simulink model "power_PVarray_islanding_detection"  (R2020a)
settings: Solver=VariableStepAuto  StartTime=0.0  StopTime=Simulation_Time  RelTol=1e-3
values from neighbouring files (symbols this model uses):
  Dinit = 0.5    [power_PVarray_100kW_param.m]
  Fnom = 60    [power_PVarray_100kW_param.m]
  Increment_MPPT = 0.01    [power_PVarray_100kW_param.m]
  Limits_MPPT = [ 1 0 ]    [power_PVarray_100kW_param.m]
  Pnom = 100e3    (= 100000)    [power_PVarray_100kW_param.m]
  Ts_Control = 10*Ts_Power    (= 5.05050505051e-05)    [power_PVarray_100kW_param.m]
  Ts_Power = 1/(33*Fnom)/100    (= 5.05050505051e-06)    [power_PVarray_100kW_param.m]
undefined symbols (not defined in the file or in its folder): D1, Delta
libraries: powerlib x29, powerlib_meascontrol x14, simulink x2, re_lib x1
(part 1 of 2)
settings Model: Creator=jfgf1  LastModifiedBy=jfgf1
settings DataIOCC: ReturnWorkspaceOutputs=off

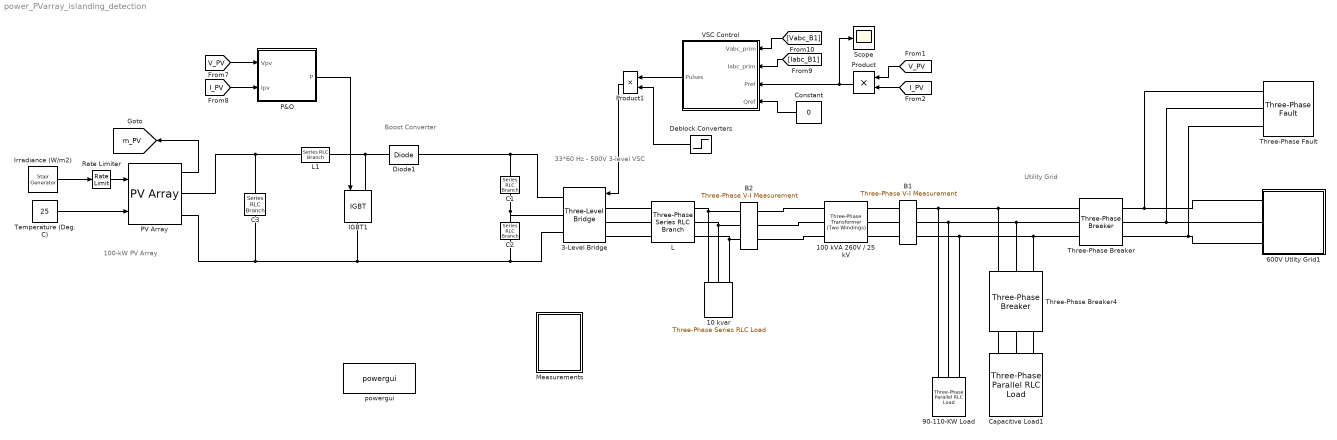
== system power_PVarray_islanding_detection ==
  note: Boost Converter
  note: 33*60 Hz - 500V
      | 3-level VSC
  note: 100-kW PV Array
  note: Utility Grid
  10 kvar : powerlib/Elements/Three-Phase Series RLC Load  LConnTagsString=A|B|C  Configuration=Y (grounded)  NominalVoltage=Vnom_dc  Vabc=[1e3 1e3 1e3]  Vabcp=[1e3 1e3 1e3]  NominalFrequency=Fnom  UnbalancedPower=off  ActivePower=10e3/100  InductivePower=0  CapacitivePower=10e3  Pabc=[10e3 9e3 11e3]  QLabc=[100 90 110]  QCabc=[100 90 110]  Pabcp=[10e3 9e3 11e3]  QLabcp=[100 90 110]  QCabcp=[100 90 110]  Measurements=None  LoadType=constant Z
  100 kVA 260V / 25 kV : powerlib/Elements/Three-Phase Transformer (Two Windings)  Winding1Connection=Yg  Winding2Connection=Delta (D1)  CoreType=Three single-phase transformers  SetSaturation=off  Hysteresis=off  DataFile='hysteresis'  SetInitialFlux=off  Measurements=None  UNITS=pu  NominalPower=[100e3 , 60 ]  Winding1=[ 25e3 , 0.001 , 0.03 ]  Winding2=[ 260 , 0.001 , 0.03 ]  Rm=500  Lm=500  L0=0.5  Saturation=[ 0,0 ; 0.0024,1.2 ; 1.0,1.52 ]  InitialFluxes=[ 0.8 , -0.8 , 0.7 ]  BreakLoop=off  DiscreteSolver=Trapezoidal iterative  DataType=off  TransfoNumber=0
  3-Level Bridge : powerlib/Power Electronics/Three-Level Bridge  Arms=3  SnubberResistance=1e6  SbubberCapacitance=inf  Device=IGBT / Diodes  Ron=0.2e-3  ForwardVoltages="[  0  0 ]"  Measurements=None
      settings: SourceProductBaseCode=PS
  600V Utlity Grid1 : Subsystem
      mask Display: image(imread('grid.jpg'))
  90-110-KW Load : powerlib/Elements/Three-Phase Parallel RLC Load  LConnTagsString=A|B|C  Configuration=Y (grounded)  NominalVoltage=Vnom_prim  Vabc=[1e3 1e3 1e3]  Vabcp=[1e3 1e3 1e3]  NominalFrequency=Fnom  UnbalancedPower=off  ActivePower=activeP  InductivePower=0  CapacitivePower=0  Pabc=[10e3 9e3 11e3]  QLabc=[100 90 110]  QCabc=[100 90 110]  Pabcp=[10e3 9e3 11e3]  QLabcp=[100 90 110]  QCabcp=[100 90 110]  Measurements=None  LoadType=constant Z
  B1 : powerlib/Measurements/Three-Phase V-I Measurement  VoltageMeasurement=phase-to-ground  SetLabelV=on  LabelV=Vabc_B1  Vpu=off  VpuLL=off  CurrentMeasurement=yes  SetLabelI=on  LabelI=Iabc_B1  Ipu=off  Pbase=100e6  Vbase=500e3  OutputType=Magnitude  PhasorSimulation=off  PSBequivalent=0
  B2 : powerlib/Measurements/Three-Phase V-I Measurement  VoltageMeasurement=phase-to-ground  SetLabelV=on  LabelV=Vabc  Vpu=off  VpuLL=off  CurrentMeasurement=no  SetLabelI=off  LabelI=Iabc  Ipu=off  Pbase=100e6  Vbase=500e3  OutputType=Magnitude  PhasorSimulation=off  PSBequivalent=0
  C1 : powerlib/Elements/Series RLC Branch  LConnTagsString=__new0  RConnTagsString=__new0  BranchType=C  Resistance=1.0  Inductance=1.0  SetiL0=off  InitialCurrent=0  Capacitance=12000e-06  Setx0=off  InitialVoltage=0  Measurements=None
  C2 : powerlib/Elements/Series RLC Branch  LConnTagsString=__new0  RConnTagsString=__new0  BranchType=C  Resistance=1.0  Inductance=1.0  SetiL0=off  InitialCurrent=0  Capacitance=12000e-06  Setx0=off  InitialVoltage=0  Measurements=None
  C3 : powerlib/Elements/Series RLC Branch  LConnTagsString=__new0  RConnTagsString=__new0  BranchType=C  Resistance=1.0  Inductance=1.0  SetiL0=off  InitialCurrent=0  Capacitance=100e-6  Setx0=off  InitialVoltage=0  Measurements=Branch voltage
  Capacitive Load1 : powerlib/Elements/Three-Phase Parallel RLC Load  LConnTagsString=A|B|C  Configuration=Y (grounded)  NominalVoltage=Vnom_prim  Vabc=[1e3 1e3 1e3]  Vabcp=[1e3 1e3 1e3]  NominalFrequency=Fnom  UnbalancedPower=off  ActivePower=0  InductivePower=0  CapacitivePower=800e3  Pabc=[10e3 9e3 11e3]  QLabc=[100 90 110]  QCabc=[100 90 110]  Pabcp=[10e3 9e3 11e3]  QLabcp=[100 90 110]  QCabcp=[100 90 110]  Measurements=None  LoadType=constant Z
  Constant : Constant  Value=0
  Deblock Converters : Step  Time=0.05  SampleTime=0
  Diode1 : powerlib/Power Electronics/Diode  Ron=1e-4  Lon=0  Vf=0  IC=0  UseSnubber=off  Rs=inf  Cs=inf  Measurements=off
  IGBT1 : powerlib/Power Electronics/IGBT  Ron=0.001  Lon=0  Vf=0  Tf=0  Tt=0  IC=0  Rs=1e5  Cs=inf  Measurements=off
  Irradiance (W/m2) : powerlib_meascontrol/Pulse & Signal Generators/Stair Generator  t=[0, 0.4, 1.0]  e=[1, 1, 1]*1000  Ts=Ts_Power
  L : powerlib/Elements/Three-Phase Series RLC Branch  LConnTagsString=A|B|C  RConnTagsString=A|B|C  BranchType=RL  Resistance=500e-6*377/50/2  Inductance=500e-6/2  Capacitance=inf  Measurements=None
  L1 : powerlib/Elements/Series RLC Branch  LConnTagsString=__new0  RConnTagsString=__new0  BranchType=RL  Resistance=0.005  Inductance=5e-3  SetiL0=off  InitialCurrent=0  Capacitance=1e-6  Setx0=off  InitialVoltage=0  Measurements=None
  Measurements : Subsystem
  P&O : Subsystem
  PV Array : re_lib/Solar/PV Array  Npar=66  Nser=5  PlotType=array @ 1000 W/m2 & specified temperatures  S_vec="[ 1000  250 ]"  Temp_C_vec="[0 25 50  ]"  ModuleName=SunPower SPR-305E-WHT-D  PlotWhenSelected=off  Pm=305.226  Ncell=96  Voc=64.2  Isc=5.96  Vm=54.7  Im=5.58  beta_Voc_pc=-0.27269  alpha_Isc_pc=0.061745  beta_Voc=-0.17507  alpha_Isc=0.00368  IL=6.0092  I0=6.3014e-12  nI=0.94504  Rsh=269.5934  Rs=0.37152  RobustModel=off  RobustCellTemperature=25  BAL=on  Tc=1e-6  Tfilter=5e-5
  Product : Product
  Product1 : Product  RndMeth=Zero
  Rate Limiter : RateLimiter  RisingSlewLimit=6000  FallingSlewLimit=-6000  SampleTimeMode=inherited  InitialCondition=1000
  Scope : Scope
  Temperature (Deg. C) : Constant  Value=25
  Three-Phase Breaker : powerlib/Elements/Three-Phase Breaker  InitialState=closed  SwitchA=on  SwitchB=on  SwitchC=on  SwitchTimes=switching_PCC  External=off  BreakerResistance=0.01  SnubberResistance=1e6  SnubberCapacitance=inf  Measurements=None
  Three-Phase Breaker4 : powerlib/Elements/Three-Phase Breaker  InitialState=closed  SwitchA=on  SwitchB=on  SwitchC=on  SwitchTimes=switching_C  External=off  BreakerResistance=0.01  SnubberResistance=800e3  SnubberCapacitance=inf  Measurements=None
  Three-Phase Fault : powerlib/Elements/Three-Phase Fault  InitialStates=0  FaultA=on  FaultB=off  FaultC=off  GroundFault=on  SwitchTimes=switching_fault  External=off  SwitchStatus=NaN  FaultResistance=0.001  GroundResistance=0.01  SnubberResistance=1e6  SnubberCapacitance=inf  Measurements=None
  VSC Control : Subsystem  mask(VSC Main Controller){nom=[ Pnom  Fnom ], Vnom=[ 25e3 260 ], Vnom_dc=500, RLxfo=[0.002  0.06 ], RLchoke=[2e-3  250e-6  ], K_VDCreg=[7  800], K_Ireg=[0.3 20], Ts=Ts_Control}
      mask prompts: nom "Nominal power and frequency [ Pnom(VA)  Fnom(Hz) ]:"; Vnom "Nominal primary and secondary voltages (Vrms LL) [ Vnom_prim   Vnom_sec ]:"; Vnom_dc "Nominal DC bus voltage (V):"; RLxfo "Total transformer leakage impedance (pu/Pnom) [ Rxfo  Lxf ]"; RLchoke "Choke impedance [ R(ohm) L(H) ]"; K_VDCreg "VDC regultator gains [ Kp  Ki ]:"; K_Ireg "Current regulator gains [ Kp  Ki ]:"; Ts "Sample time"
      mask init:
      | Pnom=nom(1);
      | Fnom=nom(2);
      | Vnom_prim=Vnom(1);
      | Vnom_sec=Vnom(2);
      | Zbase=Vnom_sec^2/Pnom;
      | Rtot_pu=RLxfo(1) + RLchoke(1)/Zbase;
      | Ltot_pu=RLxfo(2) + RLchoke(2)/(Zbase/(2*pi*Fnom));
      | Kp_VDCreg=K_VDCreg(1);
      | Ki_VDCreg=K_VDCreg(2);
      | Kp_Ireg=K_Ireg(1);
      | Ki_Ireg=K_Ireg(2);
      | Vdc_ref=Vnom_dc;
      | % Used to determine initial value of Boost Control (MPPT)
      | assignin('base','Vdc_ref_Inv',Vdc_ref);
  powergui : powerlib/powergui  Priority=1  SimulationMode=Discrete  SampleTime=1e-06  frequency=60  Iterations=50  frequencyindice=0  Pbase=100e6  ErrMax=1e-4  UnitsV=kV  UnitsW=MW  buscounter=0  FunctionMessages=off  echomessages=off  EnableUseOfTLC=off  CurrentSourceSwitches=off  DisableSnubberDevices=off  DisableRonSwitches=off  DisableVfSwitches=off  DisplayEquations=off  AutomaticDiscreteSolvers=off  SolverType=Tustin/Backward Euler (TBE)  Interpol=off  ExternalGateDelay=off  methode=off  Ts=0  x0status=blocks  SPID=off  SwTol=0  HookPort=off  NonlinearTolerance=1e-8  nMaxIteration=10  ContinueOnMaxIteration=off  RestoreLinks=warning  ResistiveCurrentMeasurement=off  Frange=[0:2:500]  Ylog=off  Xlog=on  ShowGrid=off  save=off  variable=ZData  structure=0  ZoomFFT=on  StartTime=0.0  cycles=1  DisplayStyle=1  fundamental=60  FreqAxis=off  MaxFrequency=1000  frequencyindicesteady=1  RmsSteady=1  display=off
  tag scope: m_PV=global
  wires:
  Temperature (Deg. C)/1 -> PV Array/2
  Irradiance (W/m2)/1 -> Rate Limiter/1
  PV Array/1 -> [m_PV]
  [V_PV] -> P&O/1(Vpv)
  [I_PV] -> P&O/2(Ipv)
  Constant/1 -> VSC Control/4(Qref)
  [I_PV] -> Product/2
  [V_PV] -> Product/1
  Product1/1 -> 3-Level Bridge/1
  Product/1 -> VSC Control/3(Pref), Scope/1
  [Iabc_B1] -> VSC Control/2(Iabc_prim)
  [Vabc_B1] -> VSC Control/1(Vabc_prim)
  VSC Control/1(Pulses) -> Product1/1
  Deblock Converters/1 -> Product1/2
  Rate Limiter/1 -> PV Array/1
  P&O/1(P) -> IGBT1/1
  connections:
  C3/LConn1 -- L1/LConn1 -- PV Array/RConn1
  3-Level Bridge/RConn3 -- IGBT1/RConn1 -- C3/RConn1 -- PV Array/RConn2 -- C2/RConn1
  3-Level Bridge/RConn1 -- C1/LConn1 -- Diode1/RConn1
  C2/LConn1 -- 3-Level Bridge/RConn2 -- C1/RConn1
  L1/RConn1 -- IGBT1/LConn1 -- Diode1/LConn1
  L/RConn2 -- B2/LConn2 -- 10 kvar/LConn2
  L/RConn1 -- 10 kvar/LConn1 -- B2/LConn1
  B2/LConn3 -- L/RConn3 -- 10 kvar/LConn3
  L/LConn1 -- 3-Level Bridge/LConn1
  L/LConn2 -- 3-Level Bridge/LConn2
  L/LConn3 -- 3-Level Bridge/LConn3
  100 kVA 260V / 25 kV/RConn3 -- B2/RConn3
  Three-Phase Breaker/LConn3 -- Three-Phase Breaker4/LConn3 -- 90-110-KW Load/LConn3 -- B1/RConn3
  Three-Phase Breaker/LConn1 -- Three-Phase Breaker4/LConn1 -- 90-110-KW Load/LConn1 -- B1/RConn1
  100 kVA 260V / 25 kV/RConn1 -- B2/RConn1
  Three-Phase Breaker/LConn2 -- Three-Phase Breaker4/LConn2 -- 90-110-KW Load/LConn2 -- B1/RConn2
  B1/LConn3 -- 100 kVA 260V / 25 kV/LConn3
  B1/LConn2 -- 100 kVA 260V / 25 kV/LConn2
  100 kVA 260V / 25 kV/RConn2 -- B2/RConn2
  B1/LConn1 -- 100 kVA 260V / 25 kV/LConn1
  Three-Phase Breaker/RConn1 -- Three-Phase Fault/LConn1 -- 600V Utlity Grid1/LConn1
  Three-Phase Breaker/RConn2 -- Three-Phase Fault/LConn2 -- 600V Utlity Grid1/LConn2
  Three-Phase Breaker/RConn3 -- Three-Phase Fault/LConn3 -- 600V Utlity Grid1/LConn3
  Capacitive Load1/LConn1 -- Three-Phase Breaker4/RConn1
  Three-Phase Breaker4/RConn2 -- Capacitive Load1/LConn2
  Three-Phase Breaker4/RConn3 -- Capacitive Load1/LConn3

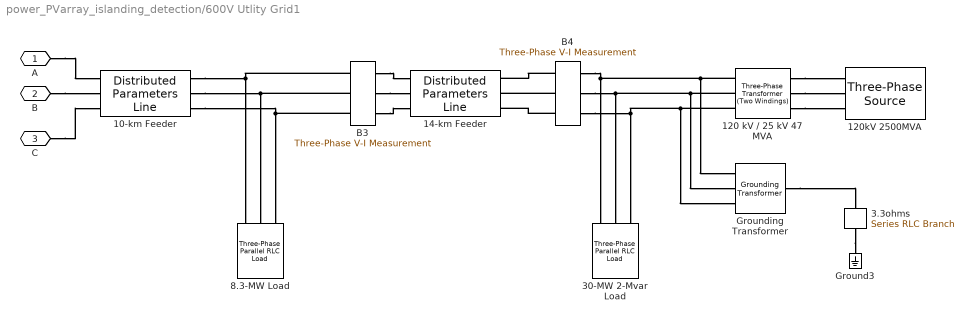
== system power_PVarray_islanding_detection/600V Utlity Grid1 ==
  10-km Feeder : powerlib/Elements/Distributed Parameters Line  Phases=3  Frequency=Fnom  Resistance=[0.1153 0.413]  Inductance=[1.05e-3 3.32e-3]  Capacitance=[11.33e-009 5.01e-009]  Length=10  x1=[-4.1e-05 1.31145391612596e-09 0 0;-4e-05 1.3127563025415e-09 0 0;-3.9e-05 1.31405850238509e-09 0 0;-3.8e-05 1.31536051547166e-09 0 0;-3.7e-05 1.31666234161617e-09 0 0;-3.6e-05 1.3179639806336e-09 0 0;-3.5e-05 1.31926543233895e-09 -5402.42576667042 -23138.0301536426;-3.4e-05 1.32056669654726e-09 -5393.70255110855 -23140.0651759113;-3.3e-05 1.3218677730736e-09 -5384.97856898125 -23142.0969094607;-3.2e-05 1.32316866173304e-09 -5376.2538215284 -23144.125354002;-3.1e-05 1.32446936234071e-09 -5367.52830998999 -23146.150509247;-3e-05 1.32576987471174e-09 -5358.8020356061 -23148.1723749077;-2.9e-05 1.32707019866131e-09 -5350.07499961693 -23150.190950697;-2.8e-05 1.32837033400461e-09 -5341.34720326278 -23152.2062363278;-2.7e-05 1.32967028055686e-09 -5332.61864778408 -23154.2182315137;-2.6e-05 1.3309700381333e-09 -5323.88933442134 -23156.2269359689;-2.5e-05 1.33226960654922e-09 -5315.1592644152 -23158.2323494078;-2.4e-05 1.33356898561992e-09 -5306.42843900638 -23160.2344715454;-2.3e-05 1.33486817516073e-09 -5297.69685943574 -23162.2333020972;-2.2e-05 1.33616717498699e-09 -5288.96452694423 -23164.2288407791;-2.1e-05 1.33746598491411e-09 -5280.23144277291 -23166.2210873075;-2e-05 1.33876460475747e-09 -5271.49760816295 -23168.2100413992;-1.9e-05 1.34006303433253e-09 -5262.76302435561 -23170.1957027716;-1.8e-05 1.34136127345475e-09 -5254.02769259227 -23172.1780711424;-1.7e-05 1.34265932193962e-09 -5245.29161411443 -23174.1571462299;-1.6e-05 1.34395717960265e-09 -5236.55479016367 -23176.1329277529;-1.5e-05 1.3452548462594e-09 -5227.81722198169 -23178.1054154305;-1.4e-05 1.34655232172543e-09 -5219.07891081029 -23180.0746089825;-1.3e-05 1.34784960581635e-09 -5210.33985789138 -23182.0405081288;-1.2e-05 1.34914669834777e-09 -5201.60006446699 -23184.0031125903;-1.1e-05 1.35044359913537e-09 -5192.85953177921 -23185.9624220878;-1e-05 1.35174030799481e-09 -5184.11826107029 -23187.918436343;-9e-06 1.3530368247418e-09 -5175.37625358255 -23189.8711550778;-8e-06 1.35433314919209e-09 -5166.63351055843 -23191.8205780148;-7e-06 1.35562928116144e-09 -5157.89003324046 -23193.7667048769;-6e-06 1.35692522046563e-09 -5149.14582287128 -23195.7095353875;-5e-06 1.35822096692048e-09 -5140.40088069365 -23197.6490692704;-4e-06 1.35951652034185e-09 -5131.65520795041 -23199.58530625;-3e-06 1.3608118805456e-09 -5122.90880588453 -23201.5182460512;-2e-06 1.36210704734763e-09 -5114.16167573905 -23203.4478883992;-1e-06 1.36340202056387e-09 -5105.41381875715 -23205.3742330198]  x2=[-4.1e-05 1.33995737415073e-09 0 0;-4e-05 1.34130776092081e-09 0 0;-3.9e-05 1.34265795706114e-09 0 0;-3.8e-05 1.34400796237984e-09 0 0;-3.7e-05 1.34535777668502e-09 0 0;-3.6e-05 1.34670739978487e-09 0 0;-3.5e-05 1.34805683148756e-09 -5385.24656512758 -23143.2120767652;-3.4e-05 1.34940607160131e-09 -5376.52139724753 -23145.2406222594;-3.3e-05 1.35075511993436e-09 -5367.79546524388 -23147.2658782988;-3.2e-05 1.35210397629498e-09 -5359.06877035679 -23149.2878445954;-3.1e-05 1.35345264049148e-09 -5350.34131382651 -23151.306520862;-3e-05 1.35480111233217e-09 -5341.61309689341 -23153.3219068116;-2.9e-05 1.35614939162541e-09 -5332.88412079796 -23155.3340021579;-2.8e-05 1.35749747817958e-09 -5324.15438678074 -23157.3428066147;-2.7e-05 1.35884537180308e-09 -5315.42389608245 -23159.3483198967;-2.6e-05 1.36019307230434e-09 -5306.69264994387 -23161.3505417188;-2.5e-05 1.36154057949184e-09 -5297.96064960593 -23163.3494717965;-2.4e-05 1.36288789317406e-09 -5289.22789630962 -23165.3451098456;-2.3e-05 1.36423501315951e-09 -5280.49439129607 -23167.3374555825;-2.2e-05 1.36558193925674e-09 -5271.7601358065 -23169.3265087242;-2.1e-05 1.36692867127433e-09 -5263.02513108225 -23171.3122689878;-2e-05 1.36827520902086e-09 -5254.28937836475 -23173.2947360912;-1.9e-05 1.36962155230498e-09 -5245.55287889556 -23175.2739097525;-1.8e-05 1.37096770093532e-09 -5236.81563391631 -23177.2497896907;-1.7e-05 1.37231365472058e-09 -5228.07764466877 -23179.2223756247;-1.6e-05 1.37365941346947e-09 -5219.33891239481 -23181.1916672743;-1.5e-05 1.37500497699072e-09 -5210.59943833638 -23183.1576643596;-1.4e-05 1.37635034509309e-09 -5201.85922373557 -23185.1203666012;-1.3e-05 1.37769551758539e-09 -5193.11826983455 -23187.07977372;-1.2e-05 1.37904049427643e-09 -5184.37657787562 -23189.0358854378;-1.1e-05 1.38038527497506e-09 -5175.63414910114 -23190.9887014764;-1e-05 1.38172985949015e-09 -5166.89098475364 -23192.9382215583;-9e-06 1.38307424763062e-09 -5158.14708607569 -23194.8844454064;-8e-06 1.38441843920539e-09 -5149.40245431 -23196.8273727442;-7e-06 1.38576243402343e-09 -5140.65709069939 -23198.7670032954;-6e-06 1.38710623189373e-09 -5131.91099648676 -23200.7033367845;-5e-06 1.38844983262529e-09 -5123.16417291513 -23202.6363729363;-4e-06 1.38979323602716e-09 -5114.41662122761 -23204.5661114759;-3e-06 1.39113644190842e-09 -5105.66834266743 -23206.4925521292;-2e-06 1.39247945007817e-09 -5096.91933847791 -23208.4156946224;-1e-06 1.39382226034554e-09 -5088.16960990249 -23210.3355386821]  x3=[-4.1e-05 -6.52349176014467e-12 0 0;-4e-05 -6.52032398932471e-12 0 0;-3.9e-05 -6.5171552918213e-12 0 0;-3.8e-05 -6.51398566808478e-12 0 0;-3.7e-05 -6.51081511856562e-12 0 0;-3.6e-05 -6.50764364371443e-12 0 0;-3.5e-05 -6.50447124398195e-12 -18.2306561580198 -80.0189566853611;-3.4e-05 -6.50129791981904e-12 -18.2004884272665 -80.0258237944139;-3.3e-05 -6.49812367167671e-12 -18.1703181098179 -80.0326795300124;-3.2e-05 -6.49494850000609e-12 -18.1401452099618 -80.0395238911823;-3.1e-05 -6.49177240525843e-12 -18.1099697319866 -80.0463568769508;-3e-05 -6.48859538788514e-12 -18.0797916801808 -80.0531784863469;-2.9e-05 -6.48541744833774e-12 -18.0496110588333 -80.0599887184009;-2.8e-05 -6.48223858706789e-12 -18.0194278722336 -80.0667875721451;-2.7e-05 -6.47905880452736e-12 -17.9892421246714 -80.0735750466132;-2.6e-05 -6.47587810116809e-12 -17.9590538204366 -80.0803511408404;-2.5e-05 -6.47269647744211e-12 -17.9288629638198 -80.0871158538639;-2.4e-05 -6.46951393380161e-12 -17.8986695591117 -80.0938691847221;-2.3e-05 -6.4663304706989e-12 -17.8684736106034 -80.1006111324552;-2.2e-05 -6.46314608858642e-12 -17.8382751225866 -80.1073416961052;-2.1e-05 -6.45996078791675e-12 -17.8080740993531 -80.1140608747153;-2e-05 -6.45677456914257e-12 -17.7778705451951 -80.1207686673307;-1.9e-05 -6.45358743271674e-12 -17.7476644644052 -80.1274650729981;-1.8e-05 -6.4503993790922e-12 -17.7174558612764 -80.1341500907657;-1.7e-05 -6.44721040872206e-12 -17.687244740102 -80.1408237196834;-1.6e-05 -6.44402052205953e-12 -17.6570311051756 -80.1474859588029;-1.5e-05 -6.44082971955798e-12 -17.6268149607914 -80.1541368071771;-1.4e-05 -6.43763800167088e-12 -17.5965963112436 -80.1607762638609;-1.3e-05 -6.43444536885185e-12 -17.566375160827 -80.1674043279107;-1.2e-05 -6.43125182155463e-12 -17.5361515138368 -80.1740209983845;-1.1e-05 -6.4280573602331e-12 -17.5059253745684 -80.1806262743419;-1e-05 -6.42486198534127e-12 -17.4756967473176 -80.1872201548441;-9e-06 -6.42166569733326e-12 -17.4454656363805 -80.193802638954;-8e-06 -6.41846849666335e-12 -17.4152320460537 -80.2003737257361;-7e-06 -6.41527038378591e-12 -17.384995980634 -80.2069334142565;-6e-06 -6.41207135915548e-12 -17.3547574444187 -80.2134817035829;-5e-06 -6.40887142322672e-12 -17.3245164417053 -80.2200185927847;-4e-06 -6.40567057645439e-12 -17.2942729767918 -80.2265440809328;-3e-06 -6.40246881929342e-12 -17.2640270539763 -80.2330581670998;-2e-06 -6.39926615219885e-12 -17.2337786775576 -80.2395608503598;-1e-06 -6.39606257562584e-12 -17.2035278518347 -80.2460521297888]  x4=[-4.1e-05 1.05357842266867e-11 0 0;-4e-05 1.05355469230034e-11 0 0;-3.9e-05 1.05353081219839e-11 0 0;-3.8e-05 1.05350678236622e-11 0 0;-3.7e-05 1.05348260280724e-11 0 0;-3.6e-05 1.05345827352489e-11 0 0;-3.5e-05 1.05343379452263e-11 -18.0916660851199 -71.3485155916182;-3.4e-05 1.05340916580393e-11 -18.0647670434512 -71.3553309187807;-3.3e-05 1.05338438737229e-11 -18.0378654343762 -71.3621361047593;-3.2e-05 1.05335945923124e-11 -18.0109612617182 -71.368931148587;-3.1e-05 1.05333438138432e-11 -17.984054529301 -71.3757160492978;-3e-05 1.05330915383509e-11 -17.9571452409485 -71.3824908059276;-2.9e-05 1.05328377658714e-11 -17.9302334004853 -71.3892554175135;-2.8e-05 1.05325824964408e-11 -17.903319011736 -71.3960098830941;-2.7e-05 1.05323257300953e-11 -17.8764020785258 -71.4027542017095;-2.6e-05 1.05320674668714e-11 -17.8494826046801 -71.409488372401;-2.5e-05 1.05318077068058e-11 -17.822560594025 -71.4162123942117;-2.4e-05 1.05315464499355e-11 -17.7956360503865 -71.422926266186;-2.3e-05 1.05312836962976e-11 -17.7687089775912 -71.4296299873696;-2.2e-05 1.05310194459294e-11 -17.7417793794661 -71.4363235568097;-2.1e-05 1.05307536988685e-11 -17.7148472598385 -71.4430069735551;-2e-05 1.05304864551526e-11 -17.6879126225361 -71.4496802366559;-1.9e-05 1.05302177148197e-11 -17.6609754713868 -71.4563433451637;-1.8e-05 1.05299474779081e-11 -17.634035810219 -71.4629962981316;-1.7e-05 1.05296757444561e-11 -17.6070936428614 -71.4696390946139;-1.6e-05 1.05294025145023e-11 -17.5801489731432 -71.4762717336666;-1.5e-05 1.05291277880857e-11 -17.5532018048937 -71.482894214347;-1.4e-05 1.05288515652451e-11 -17.5262521419428 -71.489506535714;-1.3e-05 1.05285738460199e-11 -17.4992999881206 -71.4961086968278;-1.2e-05 1.05282946304496e-11 -17.4723453472576 -71.50270069675;-1.1e-05 1.05280139185738e-11 -17.4453882231846 -71.5092825345439;-1e-05 1.05277317104325e-11 -17.418428619733 -71.5158542092739;-9e-06 1.05274480060657e-11 -17.3914665407341 -71.5224157200061;-8e-06 1.05271628055137e-11 -17.36450199002 -71.5289670658079;-7e-06 1.05268761088171e-11 -17.337534971423 -71.5355082457484;-6e-06 1.05265879160167e-11 -17.3105654887755 -71.5420392588977;-5e-06 1.05262982271534e-11 -17.2835935459107 -71.5485601043278;-4e-06 1.05260070422683e-11 -17.2566191466617 -71.5550707811118;-3e-06 1.05257143614029e-11 -17.2296422948623 -71.5615712883244;-2e-06 1.05254201845987e-11 -17.2026629943465 -71.5680616250419;-1e-06 1.05251245118976e-11 -17.1756812489486 -71.5745417903416]  x5=4.0783820321299e-05  V1=[0 0 0 7.655e-09 2.411e+04 2.411e+04;0 0 0 377 377 377;1.571 1.571 1.571 -2.646 -0.2338 -1.805]  V2=[0 0 0 7.796e-09 2.399e+04 2.399e+04;0 0 0 377 377 377;1.571 1.571 1.571 -2.649 -0.2317 -1.803]  I1=[0 0 0 1.571e-11 88.21 88.21;0 0 0 377 377 377;1.571 1.571 1.571 2.839 0.1284 -1.442]  I2=[0 0 0 1.332e-11 81.66 81.66;0 0 0 377 377 377;1.571 1.571 1.571 -1.715 -0.638 -2.209]  nHarmo=2  Measurements=None
  120 kV / 25 kV 47 MVA : powerlib/Elements/Three-Phase Transformer (Two Windings)  Winding1Connection=Yg  Winding2Connection=Delta (D1)  CoreType=Three single-phase transformers  SetSaturation=off  Hysteresis=off  DataFile='basic_model'  SetInitialFlux=off  Measurements=None  UNITS=pu  NominalPower=[47e6 60 ]  Winding1="[ 120e3  0.08/30   0.08 ]"  Winding2="[ 25e3  0.08/30  0.08]"  Rm=500  Lm=500  L0=0.5  Saturation="[ 0,0  ;  0.005,1.2  ;  1.0,1.4 ]"  InitialFluxes=[ 0.8 , -0.8 , 0.7 ]  BreakLoop=off  DiscreteSolver=Trapezoidal iterative  DataType=off  TransfoNumber=0
  120kV 2500MVA : powerlib/Electrical Sources/Three-Phase Source  InternalConnection=Yg  VoltagePhases=off  Voltage=120e3  PhaseAngle=0  Voltage_phases=[25e3 25e3 25e3]/sqrt(3)  PhaseAngles_phases=[0 -120 +120]  Frequency=Fnom  NonIdealSource=on  SpecifyImpedance=on  Resistance=0.8929  Inductance=16.58e-3  ShortCircuitLevel=2500e6  BaseVoltage=120e3  XRratio=7  BusType=swing  Pref=0  Qref=0  Prefabc=[10e3, 10e3, 10e3]  Qrefabc=[0, 0, 0]  Qmin=-inf  Qmax=inf
  14-km Feeder : powerlib/Elements/Distributed Parameters Line  Phases=3  Frequency=Fnom  Resistance=[0.1153 0.413]  Inductance=[1.05e-3 3.32e-3]  Capacitance=[11.33e-009 5.01e-009]  Length=14  x1=[-5.8e-05 1.31605259900835e-09 0 0;-5.7e-05 1.31740636106194e-09 0 0;-5.6e-05 1.3187599358827e-09 0 0;-5.5e-05 1.32011332327827e-09 0 0;-5.4e-05 1.32146652305629e-09 0 0;-5.3e-05 1.32281953502445e-09 0 0;-5.2e-05 1.32417235899045e-09 0 0;-5.1e-05 1.32552499476203e-09 0 0;-5e-05 1.32687744214694e-09 0 0;-4.9e-05 1.32822970095298e-09 -5507.3179882465 -23114.4672093839;-4.8e-05 1.32958177098796e-09 -5498.60364825136 -23116.541776762;-4.7e-05 1.33093365205971e-09 -5489.88852678202 -23118.613058764;-4.6e-05 1.33228534397611e-09 -5481.17262507708 -23120.6810550955;-4.5e-05 1.33363684654505e-09 -5472.45594437527 -23122.7457654626;-4.4e-05 1.33498815957446e-09 -5463.73848591543 -23124.8071895718;-4.3e-05 1.33633928287227e-09 -5455.02025093649 -23126.8653271303;-4.2e-05 1.33769021624647e-09 -5446.30124067753 -23128.9201778453;-4.1e-05 1.33904095950505e-09 -5437.58145637769 -23130.9717414251;-4e-05 1.34039151245606e-09 -5428.86089927627 -23133.0200175778;-3.9e-05 1.34174187490753e-09 -5420.13957061263 -23135.0650060125;-3.8e-05 1.34309204666756e-09 -5411.41747162629 -23137.1067064386;-3.7e-05 1.34444202754426e-09 -5402.69460355684 -23139.1451185657;-3.6e-05 1.34579181734577e-09 -5393.97096764399 -23141.1802421044;-3.5e-05 1.34714141588024e-09 -5385.24656512758 -23143.2120767652;-3.4e-05 1.34849082295587e-09 -5376.52139724753 -23145.2406222594;-3.3e-05 1.34984003838089e-09 -5367.79546524388 -23147.2658782988;-3.2e-05 1.35118906196353e-09 -5359.06877035679 -23149.2878445954;-3.1e-05 1.35253789351207e-09 -5350.34131382651 -23151.306520862;-3e-05 1.35388653283481e-09 -5341.61309689341 -23153.3219068116;-2.9e-05 1.35523497974009e-09 -5332.88412079796 -23155.3340021579;-2.8e-05 1.35658323403624e-09 -5324.15438678074 -23157.3428066147;-2.7e-05 1.35793129553167e-09 -5315.42389608245 -23159.3483198967;-2.6e-05 1.35927916403478e-09 -5306.69264994387 -23161.3505417188;-2.5e-05 1.360626839354e-09 -5297.96064960593 -23163.3494717965;-2.4e-05 1.3619743212978e-09 -5289.22789630962 -23165.3451098456;-2.3e-05 1.36332160967468e-09 -5280.49439129607 -23167.3374555825;-2.2e-05 1.36466870429315e-09 -5271.7601358065 -23169.3265087242;-2.1e-05 1.36601560496177e-09 -5263.02513108225 -23171.3122689878;-2e-05 1.3673623114891e-09 -5254.28937836475 -23173.2947360912;-1.9e-05 1.36870882368376e-09 -5245.55287889556 -23175.2739097525;-1.8e-05 1.37005514135436e-09 -5236.81563391631 -23177.2497896907;-1.7e-05 1.37140126430958e-09 -5228.07764466877 -23179.2223756247;-1.6e-05 1.37274719235809e-09 -5219.33891239481 -23181.1916672743;-1.5e-05 1.37409292530862e-09 -5210.59943833638 -23183.1576643596;-1.4e-05 1.37543846296989e-09 -5201.85922373557 -23185.1203666012;-1.3e-05 1.37678380515068e-09 -5193.11826983455 -23187.07977372;-1.2e-05 1.37812895165979e-09 -5184.37657787562 -23189.0358854378;-1.1e-05 1.37947390230604e-09 -5175.63414910114 -23190.9887014764;-1e-05 1.38081865689828e-09 -5166.89098475364 -23192.9382215583;-9e-06 1.3821632152454e-09 -5158.14708607569 -23194.8844454064;-8e-06 1.3835075771563e-09 -5149.40245431 -23196.8273727442;-7e-06 1.38485174243992e-09 -5140.65709069939 -23198.7670032954;-6e-06 1.38619571090522e-09 -5131.91099648676 -23200.7033367845;-5e-06 1.3875394823612e-09 -5123.16417291513 -23202.6363729363;-4e-06 1.38888305661687e-09 -5114.41662122761 -23204.5661114759;-3e-06 1.39022643348129e-09 -5105.66834266743 -23206.4925521292;-2e-06 1.39156961276353e-09 -5096.91933847791 -23208.4156946224;-1e-06 1.39291259427268e-09 -5088.16960990249 -23210.3355386821]  x2=[-5.8e-05 2.25260683526935e-09 0 0;-5.7e-05 2.25401532245857e-09 0 0;-5.6e-05 2.25542348930195e-09 0 0;-5.5e-05 2.25683133559935e-09 0 0;-5.4e-05 2.25823886115068e-09 0 0;-5.3e-05 2.25964606575591e-09 0 0;-5.2e-05 2.26105294921504e-09 0 0;-5.1e-05 2.26245951132812e-09 0 0;-5e-05 2.26386575189524e-09 0 0;-4.9e-05 2.26527167071656e-09 -3896.85585223855 -24016.4611431425;-4.8e-05 2.26667726759225e-09 -3887.80158299085 -24017.9285165165;-4.7e-05 2.26808254232255e-09 -3878.74676119984 -24019.3924764071;-4.6e-05 2.26948749470774e-09 -3869.69138815242 -24020.8530226064;-4.5e-05 2.27089212454814e-09 -3860.63546513555 -24022.3101549068;-4.4e-05 2.27229643164413e-09 -3851.57899343628 -24023.7638731012;-4.3e-05 2.27370041579612e-09 -3842.52197434174 -24025.2141769829;-4.2e-05 2.27510407680457e-09 -3833.46440913913 -24026.661066346;-4.1e-05 2.27650741446999e-09 -3824.40629911574 -24028.1045409846;-4e-05 2.27791042859294e-09 -3815.34764555892 -24029.5446006937;-3.9e-05 2.27931311897402e-09 -3806.28844975611 -24030.9812452687;-3.8e-05 2.28071548541387e-09 -3797.22871299482 -24032.4144745052;-3.7e-05 2.28211752771319e-09 -3788.16843656266 -24033.8442881997;-3.6e-05 2.28351924567271e-09 -3779.10762174727 -24035.270686149;-3.5e-05 2.28492063909322e-09 -3770.04626983641 -24036.6936681502;-3.4e-05 2.28632170777554e-09 -3760.9843821179 -24038.1132340012;-3.3e-05 2.28772245152057e-09 -3751.92195987963 -24039.5293835003;-3.2e-05 2.28912287012921e-09 -3742.85900440957 -24040.9421164461;-3.1e-05 2.29052296340245e-09 -3733.79551699578 -24042.3514326378;-3e-05 2.29192273114129e-09 -3724.73149892638 -24043.7573318753;-2.9e-05 2.29332217314679e-09 -3715.66695148956 -24045.1598139586;-2.8e-05 2.29472128922007e-09 -3706.6018759736 -24046.5588786884;-2.7e-05 2.29612007916228e-09 -3697.53627366686 -24047.954525866;-2.6e-05 2.29751854277461e-09 -3688.47014585774 -24049.3467552929;-2.5e-05 2.29891667985832e-09 -3679.40349383476 -24050.7355667713;-2.4e-05 2.30031449021471e-09 -3670.33631888649 -24052.1209601038;-2.3e-05 2.3017119736451e-09 -3661.26862230157 -24053.5029350935;-2.2e-05 2.30310912995089e-09 -3652.20040536873 -24054.881491544;-2.1e-05 2.30450595893351e-09 -3643.13166937676 -24056.2566292593;-2e-05 2.30590246039444e-09 -3634.06241561453 -24057.6283480442;-1.9e-05 2.3072986341352e-09 -3624.99264537098 -24058.9966477035;-1.8e-05 2.30869447995737e-09 -3615.92235993514 -24060.3615280428;-1.7e-05 2.31008999766257e-09 -3606.85156059609 -24061.7229888681;-1.6e-05 2.31148518705245e-09 -3597.78024864299 -24063.081029986;-1.5e-05 2.31288004792875e-09 -3588.70842536509 -24064.4356512035;-1.4e-05 2.31427458009321e-09 -3579.63609205168 -24065.7868523279;-1.3e-05 2.31566878334763e-09 -3570.56324999215 -24067.1346331674;-1.2e-05 2.31706265749388e-09 -3561.48990047595 -24068.4789935303;-1.1e-05 2.31845620233386e-09 -3552.41604479262 -24069.8199332255;-1e-05 2.3198494176695e-09 -3543.34168423173 -24071.1574520625;-9e-06 2.3212423033028e-09 -3534.26682008297 -24072.4915498512;-8e-06 2.3226348590358e-09 -3525.19145363608 -24073.8222264021;-7e-06 2.32402708467059e-09 -3516.11558618086 -24075.1494815259;-6e-06 2.3254189800093e-09 -3507.0392190072 -24076.473315034;-5e-06 2.32681054485412e-09 -3497.96235340506 -24077.7937267383;-4e-06 2.32820177900726e-09 -3488.88499066446 -24079.1107164512;-3e-06 2.32959268227101e-09 -3479.80713207549 -24080.4242839854;-2e-06 2.33098325444769e-09 -3470.72877892832 -24081.7344291543;-1e-06 2.33237349533965e-09 -3461.64993251319 -24083.0411517717]  x3=[-5.8e-05 9.77969712792975e-12 0 0;-5.7e-05 9.80058033689096e-12 0 0;-5.6e-05 9.82146215297113e-12 0 0;-5.5e-05 9.8423425732025e-12 0 0;-5.4e-05 9.86322159461749e-12 0 0;-5.3e-05 9.88409921424873e-12 0 0;-5.2e-05 9.90497542912903e-12 0 0;-5.1e-05 9.92585023629143e-12 0 0;-5e-05 9.94672363276914e-12 0 0;-4.9e-05 9.9675956155956e-12 -90.5346088964957 -386.232113122669;-4.8e-05 9.98846618180443e-12 -90.3889963901512 -386.266216419227;-4.7e-05 1.00093353284295e-11 -90.2433710375146 -386.30026481874;-4.6e-05 1.00302030525047e-11 -90.0977328592823 -386.334258316372;-4.5e-05 1.00510693510644e-11 -89.9520818761529 -386.368196907289;-4.4e-05 1.0071934221143e-11 -89.8064181088265 -386.402080586668;-4.3e-05 1.00927976597751e-11 -89.6607415780053 -386.435909349695;-4.2e-05 1.01136596639956e-11 -89.5150523043932 -386.469683191561;-4.1e-05 1.01345202308395e-11 -89.3693503086958 -386.503402107465;-4e-05 1.0155379357342e-11 -89.2236356116206 -386.537066092617;-3.9e-05 1.01762370405387e-11 -89.0779082338769 -386.570675142231;-3.8e-05 1.01970932774651e-11 -88.9321681961759 -386.604229251531;-3.7e-05 1.02179480651572e-11 -88.7864155192305 -386.637728415748;-3.6e-05 1.0238801400651e-11 -88.6406502237553 -386.671172630122;-3.5e-05 1.02596532809827e-11 -88.4948723304669 -386.704561889898;-3.4e-05 1.02805037031889e-11 -88.3490818600835 -386.737896190332;-3.3e-05 1.03013526643063e-11 -88.2032788333253 -386.771175526685;-3.2e-05 1.03222001613717e-11 -88.0574632709141 -386.80439989423;-3.1e-05 1.03430461914223e-11 -87.9116351935735 -386.837569288242;-3e-05 1.03638907514953e-11 -87.765794622029 -386.870683704009;-2.9e-05 1.03847338386283e-11 -87.6199415770077 -386.903743136824;-2.8e-05 1.04055754498591e-11 -87.4740760792387 -386.936747581988;-2.7e-05 1.04264155822255e-11 -87.3281981494526 -386.969697034811;-2.6e-05 1.04472542327657e-11 -87.182307808382 -387.00259149061;-2.5e-05 1.04680913985181e-11 -87.0364050767612 -387.03543094471;-2.4e-05 1.04889270765213e-11 -86.8904899753261 -387.068215392444;-2.3e-05 1.0509761263814e-11 -86.7445625248146 -387.100944829152;-2.2e-05 1.05305939574353e-11 -86.5986227459662 -387.133619250182;-2.1e-05 1.05514251544243e-11 -86.4526706595223 -387.166238650892;-2e-05 1.05722548518204e-11 -86.3067062862258 -387.198803026645;-1.9e-05 1.05930830466634e-11 -86.1607296468215 -387.231312372812;-1.8e-05 1.06139097359931e-11 -86.014740762056 -387.263766684775;-1.7e-05 1.06347349168494e-11 -85.8687396526776 -387.296165957919;-1.6e-05 1.06555585862728e-11 -85.7227263394363 -387.328510187641;-1.5e-05 1.06763807413036e-11 -85.5767008430838 -387.360799369343;-1.4e-05 1.06972013789826e-11 -85.4306631843736 -387.393033498437;-1.3e-05 1.07180204963508e-11 -85.2846133840609 -387.425212570342;-1.2e-05 1.07388380904492e-11 -85.1385514629027 -387.457336580483;-1.1e-05 1.07596541583192e-11 -84.9924774416575 -387.489405524296;-1e-05 1.07804686970024e-11 -84.8463913410858 -387.521419397223;-9e-06 1.08012817035406e-11 -84.7002931819498 -387.553378194714;-8e-06 1.08220931749757e-11 -84.5541829850131 -387.585281912227;-7e-06 1.08429031083501e-11 -84.4080607710412 -387.617130545227;-6e-06 1.08637115007061e-11 -84.2619265608016 -387.648924089188;-5e-06 1.08845183490865e-11 -84.1157803750629 -387.680662539593;-4e-06 1.0905323650534e-11 -83.969622234596 -387.712345891929;-3e-06 1.09261274020919e-11 -83.823452160173 -387.743974141694;-2e-06 1.09469296008033e-11 -83.6772701725682 -387.775547284393;-1e-06 1.0967730243712e-11 -83.531076292557 -387.807065315538]  x4=[-5.8e-05 -5.22013038447485e-12 0 0;-5.7e-05 -5.2375749695159e-12 0 0;-5.6e-05 -5.25501881018074e-12 0 0;-5.5e-05 -5.27246190399021e-12 0 0;-5.4e-05 -5.28990424846526e-12 0 0;-5.3e-05 -5.30734584112694e-12 0 0;-5.2e-05 -5.32478667949642e-12 0 0;-5.1e-05 -5.34222676109495e-12 0 0;-5e-05 -5.35966608344392e-12 0 0;-4.9e-05 -5.37710464406482e-12 58.360070334798 232.30717909782;-4.8e-05 -5.39454244047922e-12 58.2724884464711 232.329163817471;-4.7e-05 -5.41197947020884e-12 58.1848982763241 232.351115517966;-4.6e-05 -5.42941573077547e-12 58.0972998368054 232.373034196185;-4.5e-05 -5.44685121970105e-12 58.0096931403648 232.394919849015;-4.4e-05 -5.46428593450759e-12 57.922078199453 232.416772473343;-4.3e-05 -5.48171987271724e-12 57.8344550265221 232.438592066065;-4.2e-05 -5.49915303185225e-12 57.7468236340254 232.460378624079;-4.1e-05 -5.51658540943496e-12 57.6591840344172 232.482132144289;-4e-05 -5.53401700298787e-12 57.5715362401531 232.503852623603;-3.9e-05 -5.55144781003353e-12 57.4838802636897 232.525540058934;-3.8e-05 -5.56887782809466e-12 57.3962161174849 232.547194447201;-3.7e-05 -5.58630705469405e-12 57.3085438139978 232.568815785325;-3.6e-05 -5.60373548735463e-12 57.2208633656885 232.590404070233;-3.5e-05 -5.62116312359942e-12 57.1331747850184 232.611959298858;-3.4e-05 -5.63858996095157e-12 57.0454780844501 232.633481468136;-3.3e-05 -5.65601599693434e-12 56.957773276447 232.654970575009;-3.2e-05 -5.67344122907109e-12 56.8700603734742 232.676426616421;-3.1e-05 -5.69086565488532e-12 56.7823393879975 232.697849589324;-3e-05 -5.70828927190062e-12 56.6946103324839 232.719239490673;-2.9e-05 -5.72571207764071e-12 56.6068732194019 232.740596317428;-2.8e-05 -5.74313406962943e-12 56.5191280612208 232.761920066553;-2.7e-05 -5.76055524539071e-12 56.4313748704111 232.783210735019;-2.6e-05 -5.77797560244861e-12 56.3436136594445 232.804468319799;-2.5e-05 -5.79539513832733e-12 56.2558444407939 232.825692817873;-2.4e-05 -5.81281385055115e-12 56.1680672269331 232.846884226223;-2.3e-05 -5.83023173664449e-12 56.0802820303374 232.868042541837;-2.2e-05 -5.84764879413188e-12 55.9924888634829 232.88916776171;-2.1e-05 -5.86506502053796e-12 55.904687738847 232.910259882838;-2e-05 -5.88248041338749e-12 55.8168786689082 232.931318902224;-1.9e-05 -5.89989497020537e-12 55.7290616661461 232.952344816875;-1.8e-05 -5.9173086885166e-12 55.6412367430416 232.973337623802;-1.7e-05 -5.9347215658463e-12 55.5534039120763 232.994297320022;-1.6e-05 -5.95213359971971e-12 55.4655631857335 233.015223902557;-1.5e-05 -5.96954478766219e-12 55.3777145764972 233.036117368431;-1.4e-05 -5.98695512719923e-12 55.2898580968526 233.056977714676;-1.3e-05 -6.00436461585642e-12 55.2019937592861 233.077804938327;-1.2e-05 -6.0217732511595e-12 55.1141215762852 233.098599036424;-1.1e-05 -6.0391810306343e-12 55.0262415603384 233.119360006012;-1e-05 -6.05658795180679e-12 54.9383537239356 233.140087844139;-9e-06 -6.07399401220306e-12 54.8504580795675 233.160782547861;-8e-06 -6.09139920934932e-12 54.762554639726 233.181444114235;-7e-06 -6.10880354077191e-12 54.6746434169043 233.202072540326;-6e-06 -6.12620700399727e-12 54.5867244235963 233.222667823202;-5e-06 -6.143609596552e-12 54.4987976722975 233.243229959935;-4e-06 -6.16101131596279e-12 54.410863175504 233.263758947604;-3e-06 -6.17841215975647e-12 54.3229209457135 233.28425478329;-2e-06 -6.19581212545999e-12 54.2349709954244 233.304717464081;-1e-06 -6.21321121060043e-12 54.1470133371364 233.325146987069]  x5=5.70973484498186e-05  V1=[0 0 0 7.795e-09 2.399e+04 2.399e+04;0 0 0 377 377 377;1.571 1.571 1.571 -2.655 -0.2369 -1.808]  V2=[0 0 0 8.76e-09 2.44e+04 2.44e+04;0 0 0 377 377 377;1.571 1.571 1.571 -2.45 -0.1615 -1.732]  I1=[0 0 0 1.141e-10 401.1 401.1;0 0 0 377 377 377;1.571 1.571 1.571 -2.74 -0.1564 -1.727]  I2=[0 0 0 9.571e-11 243.2 243.2;0 0 0 377 377 377;1.571 1.571 1.571 0.3594 3.019 1.448]  nHarmo=2  Measurements=None
  "3.3ohms " : powerlib/Elements/Series RLC Branch  LConnTagsString=__new0  RConnTagsString=__new0  BranchType=R  Resistance=3.3  Inductance=[]  SetiL0=off  InitialCurrent=0  Capacitance=[]  Setx0=off  InitialVoltage=0  Measurements=None
  30-MW 2-Mvar Load : powerlib/Elements/Three-Phase Parallel RLC Load  LConnTagsString=A|B|C  Configuration=Y (grounded)  NominalVoltage=Vnom_prim  Vabc=[1e3 1e3 1e3]  Vabcp=[1e3 1e3 1e3]  NominalFrequency=Fnom  UnbalancedPower=off  ActivePower=30e6  InductivePower=2e6  CapacitivePower=0  Pabc=[10e3 9e3 11e3]  QLabc=[100 90 110]  QCabc=[100 90 110]  Pabcp=[10e3 9e3 11e3]  QLabcp=[100 90 110]  QCabcp=[100 90 110]  Measurements=None  LoadType=constant Z
  8.3-MW Load : powerlib/Elements/Three-Phase Parallel RLC Load  LConnTagsString=A|B|C  Configuration=Y (grounded)  NominalVoltage=Vnom_prim  Vabc=[1e3 1e3 1e3]  Vabcp=[1e3 1e3 1e3]  NominalFrequency=Fnom  UnbalancedPower=off  ActivePower=8.3e6  InductivePower=0  CapacitivePower=0  Pabc=[10e3 9e3 11e3]  QLabc=[100 90 110]  QCabc=[100 90 110]  Pabcp=[10e3 9e3 11e3]  QLabcp=[100 90 110]  QCabcp=[100 90 110]  Measurements=None  LoadType=constant Z
  B3 : powerlib/Measurements/Three-Phase V-I Measurement  VoltageMeasurement=phase-to-ground  SetLabelV=on  LabelV=Vabc2  Vpu=off  VpuLL=off  CurrentMeasurement=no  SetLabelI=on  LabelI=Iabc2  Ipu=off  Pbase=100e6  Vbase=500e3  OutputType=Magnitude  PhasorSimulation=off  PSBequivalent=0
  B4 : powerlib/Measurements/Three-Phase V-I Measurement  VoltageMeasurement=phase-to-ground  SetLabelV=on  LabelV=Vabc3  Vpu=off  VpuLL=off  CurrentMeasurement=no  SetLabelI=on  LabelI=Iabc3  Ipu=off  Pbase=100e6  Vbase=500e3  OutputType=Magnitude  PhasorSimulation=off  PSBequivalent=0
  Ground3 : powerlib/Elements/Ground  LConnTagsString=a
  "Grounding Transformer " : powerlib/Elements/Grounding Transformer   UNITS=pu  NominalPower="[100e6   Fnom]"  NominalVoltage=Vnom_prim  ZeroSequenceImpedance_pu=[0.025 0.75]  MagnetizationBranch_pu=[500 500]  ZeroSequenceImpedance_SI=[0.052083 589.05]  MagnetizationBranch_SI=[1041.7 3.927e+005]  Measurements=None
      settings: SourceProductBaseCode=PS
  A : PMIOPort  Side=Left
  B : PMIOPort  Port=2  Side=Left
  C : PMIOPort  Port=3  Side=Left
  connections:
  "Grounding Transformer "/RConn1 -- "3.3ohms "/LConn1
  C/RConn1 -- 10-km Feeder/LConn3
  B/RConn1 -- 10-km Feeder/LConn2
  A/RConn1 -- 10-km Feeder/LConn1
  10-km Feeder/RConn3 -- B3/LConn3 -- 8.3-MW Load/LConn3
  10-km Feeder/RConn2 -- 8.3-MW Load/LConn2 -- B3/LConn2
  10-km Feeder/RConn1 -- 8.3-MW Load/LConn1 -- B3/LConn1
  "Grounding Transformer "/LConn3 -- 120 kV / 25 kV 47 MVA/RConn3 -- B4/RConn3 -- 30-MW 2-Mvar Load/LConn3
  "Grounding Transformer "/LConn2 -- 120 kV / 25 kV 47 MVA/RConn2 -- B4/RConn2 -- 30-MW 2-Mvar Load/LConn2
  "Grounding Transformer "/LConn1 -- 120 kV / 25 kV 47 MVA/RConn1 -- 30-MW 2-Mvar Load/LConn1 -- B4/RConn1
  120 kV / 25 kV 47 MVA/LConn3 -- 120kV 2500MVA/RConn3
  120 kV / 25 kV 47 MVA/LConn2 -- 120kV 2500MVA/RConn2
  120 kV / 25 kV 47 MVA/LConn1 -- 120kV 2500MVA/RConn1
  "3.3ohms "/RConn1 -- Ground3/LConn1
  B3/RConn3 -- 14-km Feeder/LConn3
  B3/RConn1 -- 14-km Feeder/LConn1
  B3/RConn2 -- 14-km Feeder/LConn2
  B4/LConn2 -- 14-km Feeder/RConn2
  B4/LConn3 -- 14-km Feeder/RConn3
  B4/LConn1 -- 14-km Feeder/RConn1

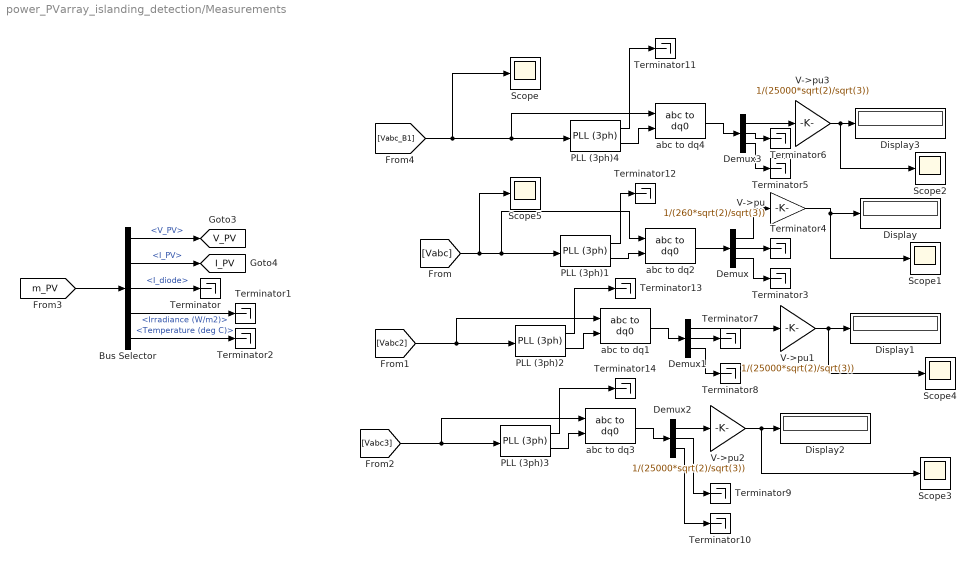
== system power_PVarray_islanding_detection/Measurements ==
  Bus Selector : BusSelector  OutputSignals=V_PV,I_PV,I_diode,Irradiance (W/m2),Temperature (deg C)
  Demux{,1..3} (4 alike) : Demux  Outputs=3
  Display{,1..3} (4 alike) : Display
  PLL (3ph){1..4} (4 alike) : powerlib_meascontrol/PLL/PLL (3ph)  Fmin=45  Par_Init="[-0.57  60]"  ParK=[180, 3200, 1]  TcD=1e-4  MaxRateChangeFreq=12  FilterCutOffFreq=25  Ts=Ts_Control  AGC=on
  Scope{,1..5} (6 alike) : Scope
  Terminator{,1..14} (15 alike) : Terminator
  V->pu : Gain  Gain=1/(260*sqrt(2)/sqrt(3))  SaturateOnIntegerOverflow=on  OutDataTypeStr=Inherit: Same as input  ParamDataTypeStr=Inherit: Same as input
  V->pu1 : Gain  Gain=1/(25000*sqrt(2)/sqrt(3))  SaturateOnIntegerOverflow=on  OutDataTypeStr=Inherit: Same as input  ParamDataTypeStr=Inherit: Same as input
  V->pu2 : Gain  Gain=1/(25000*sqrt(2)/sqrt(3))  SaturateOnIntegerOverflow=on  OutDataTypeStr=Inherit: Same as input  ParamDataTypeStr=Inherit: Same as input
  V->pu3 : Gain  Gain=1/(25000*sqrt(2)/sqrt(3))  SaturateOnIntegerOverflow=on  OutDataTypeStr=Inherit: Same as input  ParamDataTypeStr=Inherit: Same as input
  abc to dq{1..4} (4 alike) : powerlib_meascontrol/Transformations/abc to dq0  Alignment=90 degrees behind phase A axis
  tag scope: I_PV=global, V_PV=global
  wires:
  Bus Selector/3 -> Terminator/1  "<I_diode>"
  Bus Selector/1 -> [V_PV]  "<V_PV>"
  [m_PV] -> Bus Selector/1
  Bus Selector/5 -> Terminator2/1  "<Temperature (deg C)>"
  Bus Selector/4 -> Terminator1/1  "<Irradiance (W/m2)>"
  Bus Selector/2 -> [I_PV]  "<I_PV>"
  [Vabc] -> Scope5/1, abc to dq2/1, PLL (3ph)1/1
  PLL (3ph)1/2 -> abc to dq2/2
  Demux/1 -> V->pu/1
  abc to dq2/1 -> Demux/1
  V->pu/1 -> Scope1/1, Display/1
  [Vabc3] -> abc to dq3/1, PLL (3ph)3/1
  PLL (3ph)3/2 -> abc to dq3/2
  Demux2/1 -> V->pu2/1
  abc to dq3/1 -> Demux2/1
  V->pu3/1 -> Scope2/1, Display3/1
  abc to dq4/1 -> Demux3/1
  Demux3/1 -> V->pu3/1
  PLL (3ph)4/2 -> abc to dq4/2
  [Vabc_B1] -> Scope/1, PLL (3ph)4/1, abc to dq4/1
  abc to dq1/1 -> Demux1/1
  Demux1/1 -> V->pu1/1
  PLL (3ph)2/2 -> abc to dq1/2
  [Vabc2] -> PLL (3ph)2/1, abc to dq1/1
  V->pu2/1 -> Scope3/1, Display2/1
  V->pu1/1 -> Scope4/1, Display1/1
  Demux/3 -> Terminator3/1
  Demux/2 -> Terminator4/1
  Demux3/3 -> Terminator5/1
  Demux3/2 -> Terminator6/1
  Demux1/2 -> Terminator7/1
  Demux1/3 -> Terminator8/1
  Demux2/2 -> Terminator9/1
  Demux2/3 -> Terminator10/1
  PLL (3ph)4/1 -> Terminator11/1
  PLL (3ph)1/1 -> Terminator12/1
  PLL (3ph)2/1 -> Terminator13/1
  PLL (3ph)3/1 -> Terminator14/1

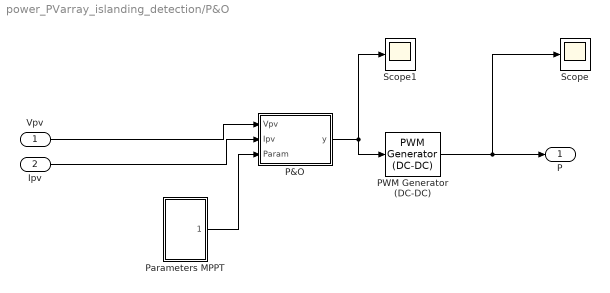
== system power_PVarray_islanding_detection/P&O ==
  Vpv : Inport
  Ipv : Inport  Port=2
  P&O : MATLAB Function  TreatAsAtomicUnit=on  SystemSampleTime=0.01
  PWM Generator (DC-DC) : powerlib_meascontrol/Pulse & Signal Generators/PWM Generator (DC-DC)  Fsw=5000  Ts=0
  Parameters MPPT : Subsystem
  Scope : Scope
  Scope1 : Scope
  P : Outport
  wires:
  P&O/1(y) -> PWM Generator (DC-DC)/1, Scope1/1
  Parameters MPPT/1(Param) -> P&O/3(Param)
  PWM Generator (DC-DC)/1 -> Scope/1, P/1
  Vpv/1 -> P&O/1(Vpv)
  Ipv/1 -> P&O/2(Ipv)

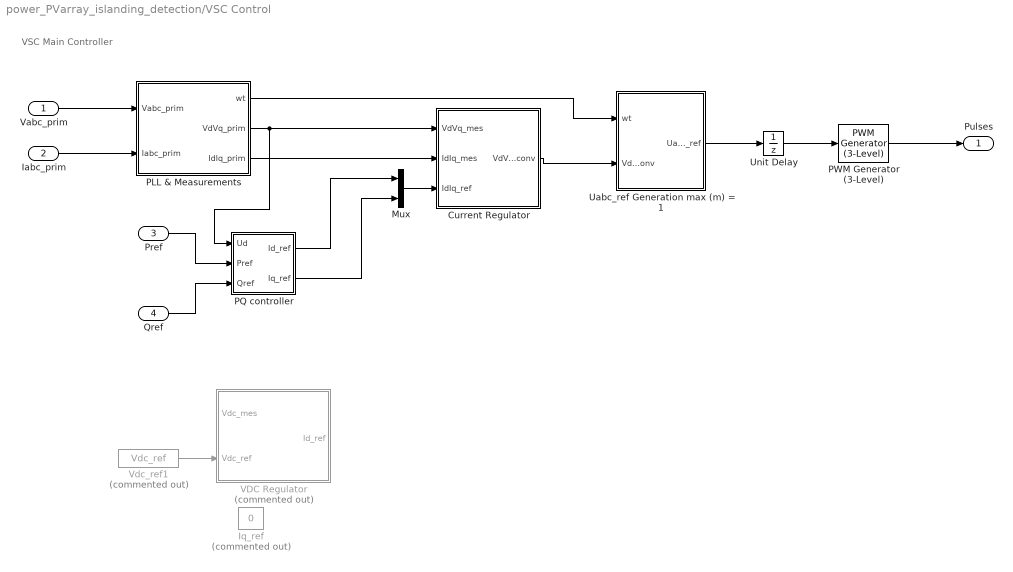
== system power_PVarray_islanding_detection/VSC Control ==
  note: VSC Main Controller
  Vabc_prim : Inport  PortDimensions=3
  Iabc_prim : Inport  Port=2  PortDimensions=3
  Pref : Inport  Port=3  PortDimensions=1
  Qref : Inport  Port=4
  Current Regulator : Subsystem
  Iq_ref : Constant  Commented=on  Value=0
  Mux : Mux  Inputs=2
  PLL & Measurements : Subsystem
  PQ controller : Subsystem
  PWM Generator (3-Level) : powerlib_meascontrol/Pulse & Signal Generators/PWM Generator (3-Level)  ModulatorType=Three-phase bridge (12 pulses)  ModulatorMode=Unsynchronized  nF=27  Fc=33*60  ModulatingSignals=off  m=0.8  Freq=60  Phase=0  Ts=Ts_Power
      settings: SourceProductBaseCode=PS
  Uabc_ref Generation max (m) = 1 : Subsystem
  Unit Delay : UnitDelay  SampleTime=Ts_Control  HasFrameUpgradeWarning=on
  VDC Regulator : Subsystem  Commented=on
  Vdc_ref1 : Constant  Commented=on  Value=Vdc_ref
  Pulses : Outport  VectorParamsAs1DForOutWhenUnconnected=off
  wires:
  PQ controller/2(Iq_ref) -> Mux/2
  PQ controller/1(Id_ref) -> Mux/1
  Qref/1 -> PQ controller/3(Qref)
  Pref/1 -> PQ controller/2(Pref)
  Vdc_ref1/1 -> VDC Regulator/2(Vdc_ref)
  Uabc_ref Generation max (m) = 1/1(Uabc_ref) -> Unit Delay/1
  PWM Generator (3-Level)/1 -> Pulses/1
  Unit Delay/1 -> PWM Generator (3-Level)/1
  Iabc_prim/1 -> PLL & Measurements/2(Iabc_prim)
  Vabc_prim/1 -> PLL & Measurements/1(Vabc_prim)
  PLL & Measurements/2(VdVq_prim) -> Current Regulator/1(VdVq_mes), PQ controller/1(Ud)
  PLL & Measurements/3(IdIq_prim) -> Current Regulator/2(IdIq_mes)
  Mux/1 -> Current Regulator/3(IdIq_ref)
  Current Regulator/1(VdVq_conv) -> Uabc_ref Generation max (m) = 1/2(VdVq_conv)
  PLL & Measurements/1(wt) -> Uabc_ref Generation max (m) = 1/1(wt)

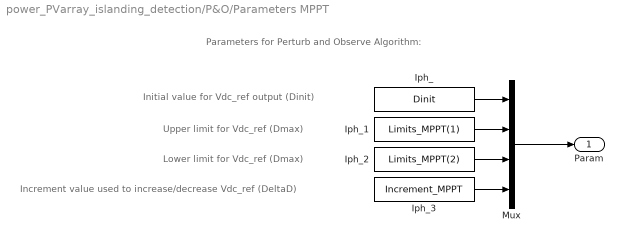
== system power_PVarray_islanding_detection/P&O/Parameters MPPT ==
  note: Upper limit for Vdc_ref (Dmax)
  note: Increment value used to increase/decrease Vdc_ref (DeltaD)
  note: Initial value for Vdc_ref output (Dinit)
  note: Parameters for Perturb and Observe Algorithm:
  note: Lower limit for Vdc_ref (Dmax)
  Iph_ : Constant  Value=Dinit
  Iph_1 : Constant  Value=Limits_MPPT(1)
  Iph_2 : Constant  Value=Limits_MPPT(2)
  Iph_3 : Constant  Value=Increment_MPPT
  Mux : Mux
  Param : Outport
  wires:
  Mux/1 -> Param/1
  Iph_3/1 -> Mux/4
  Iph_1/1 -> Mux/2
  Iph_/1 -> Mux/1
  Iph_2/1 -> Mux/3
